simulink model "Quarter_Car"  (R2018b)
settings: Solver=VariableStepAuto  StartTime=0.0  StopTime=60  RelTol=1e-3
values from neighbouring files (symbols this model uses):
  Cs = 100    [Main.m]
  Ct = 0.07    [Main.m]
  Ks = 4000    [Main.m]
  Kt = 7000    [Main.m]
  MR = 0.8    [Main.m]
  Ms = 185    [Main.m]
  Mu = 15    [Main.m]
settings Model: Creator=fcoutu3  LastModifiedBy=katlilee
settings DebuggingCC: LibraryContextMissingDiagnostic=none
settings SFSimCC: SimUseLocalCustomCode=off
settings RTWCC: RTWUseLocalCustomCode=off

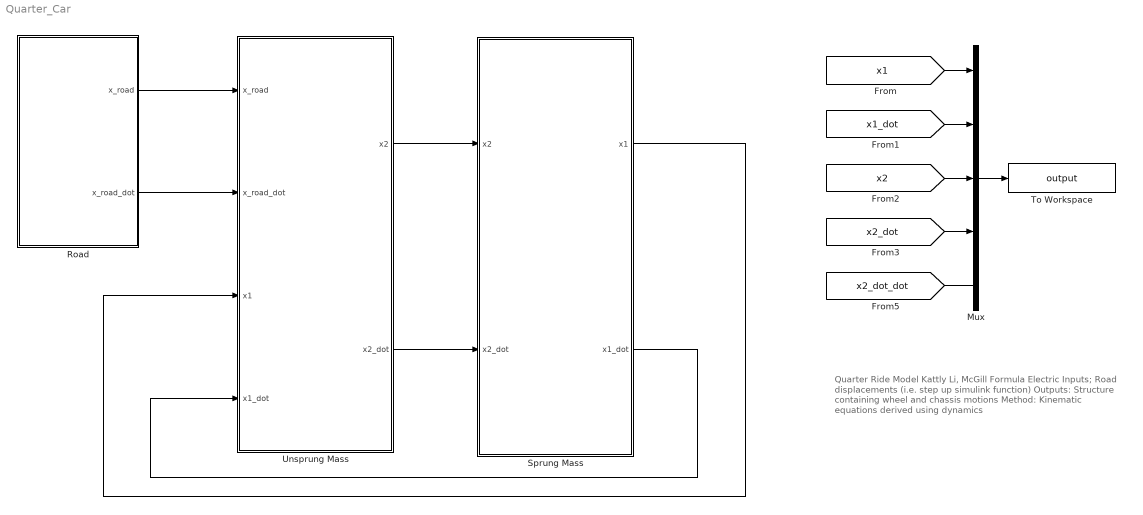
== system Quarter_Car ==
  note: Quarter Ride Model
      | Kattly Li, McGill Formula Electric
      |
      | Inputs;
      | Road displacements
      | (i.e. step up simulink function)
      |
      | Outputs:
      | Structure containing wheel and chassis motions
      |
      | Method:
      | Kinematic equations derived using dynamics
  Mux : Mux  Inputs=5
  Road : Subsystem
  Sprung Mass : Subsystem
  To Workspace : ToWorkspace  VariableName=output  SaveFormat=Structure With Time  SampleTime=-1
  Unsprung Mass : Subsystem
  wires:
  Unsprung Mass/1(x2) -> Sprung Mass/1(x2)
  Sprung Mass/1(x1) -> Unsprung Mass/3(x1)
  Unsprung Mass/2(x2_dot) -> Sprung Mass/2(x2_dot)
  Sprung Mass/2(x1_dot) -> Unsprung Mass/4(x1_dot)
  [x1_dot] -> Mux/2
  [x1] -> Mux/1
  Mux/1 -> To Workspace/1
  [x2] -> Mux/3
  [x2_dot_dot] -> ?
  Road/1(x_road) -> Unsprung Mass/1(x_road)
  Road/2(x_road_dot) -> Unsprung Mass/2(x_road_dot)
  [x2_dot] -> Mux/4

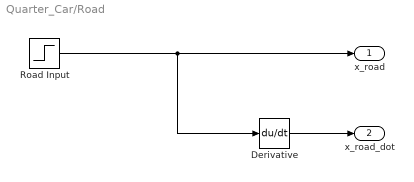
== system Quarter_Car/Road ==
  Derivative : Derivative
  Road Input : Step  After=0.01  SampleTime=0
  x_road : Outport
  x_road_dot : Outport  Port=2
  wires:
  Road Input/1 -> Derivative/1, x_road/1
  Derivative/1 -> x_road_dot/1

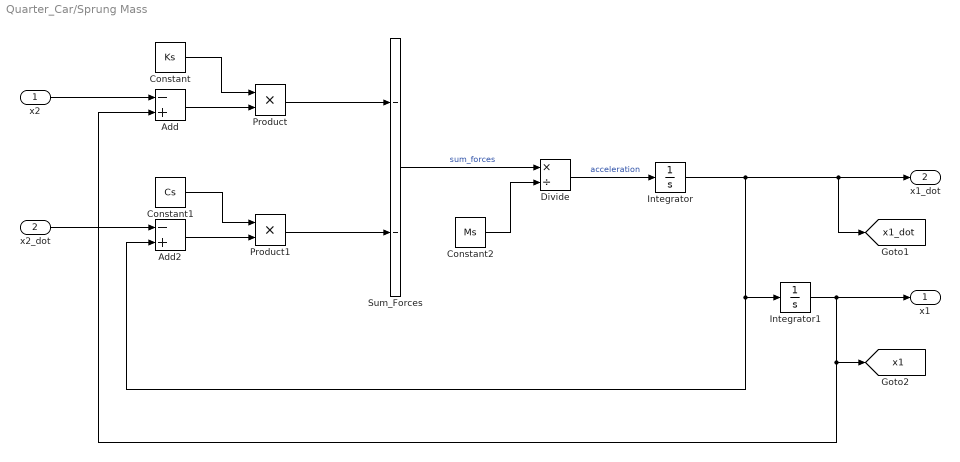
== system Quarter_Car/Sprung Mass ==
  x2 : Inport
  x2_dot : Inport  Port=2
  Add : Sum  Inputs=-+
  Add2 : Sum  Inputs=-+
  Constant : Constant  Value=Ks
  Constant1 : Constant  Value=Cs
  Constant2 : Constant  Value=Ms
  Divide : Product  Inputs=*/
  Integrator : Integrator
  Integrator1 : Integrator
  Product : Product
  Product1 : Product
  Sum_Forces : Sum  Inputs=--
  x1 : Outport
  x1_dot : Outport  Port=2
  tag scope: x1=global, x1_dot=global
  wires:
  Add/1 -> Product/2
  Product/1 -> Sum_Forces/1
  Add2/1 -> Product1/2
  Product1/1 -> Sum_Forces/2
  Constant1/1 -> Product1/1
  Sum_Forces/1 -> Divide/1  "sum_forces"
  Constant2/1 -> Divide/2
  Divide/1 -> Integrator/1  "acceleration"
  Integrator/1 -> x1_dot/1, [x1_dot], Integrator1/1, Add2/2
  Integrator1/1 -> Add/2, [x1], x1/1
  x2/1 -> Add/1
  x2_dot/1 -> Add2/1
  Constant/1 -> Product/1

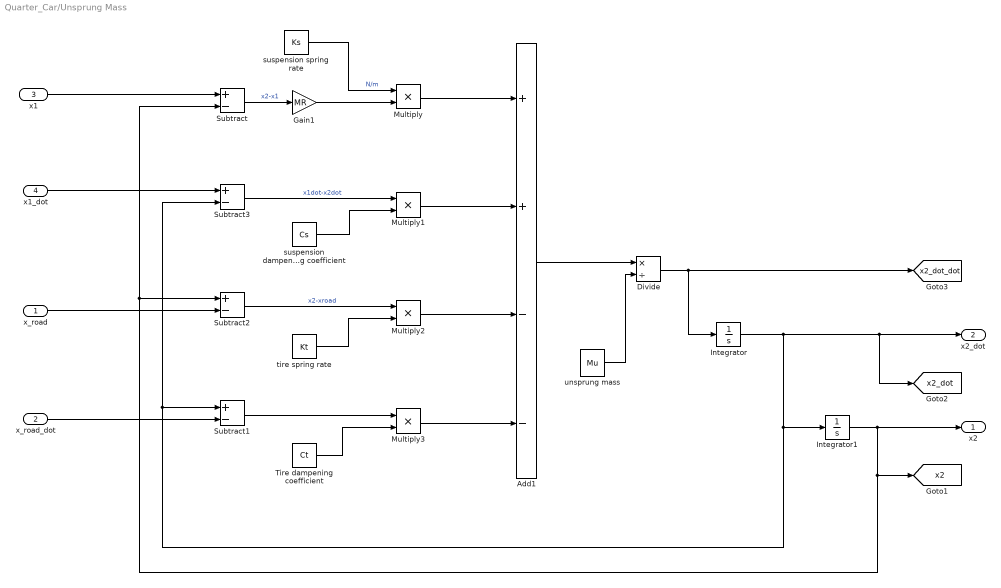
== system Quarter_Car/Unsprung Mass ==
  x_road : Inport
  x_road_dot : Inport  Port=2
  x1 : Inport  Port=3
  x1_dot : Inport  Port=4
  Add1 : Sum  Inputs=++--
  Divide : Product  Inputs=*/
  Gain1 : Gain  Gain=MR
  Integrator : Integrator
  Integrator1 : Integrator
  Multiply{,1..3} (4 alike) : Product
  Subtract{,1..3} (4 alike) : Sum  Inputs=+-
  "Tire dampening coefficient " : Constant  Value=Ct
  "suspension dampening coefficient " : Constant  Value=Cs
  "suspension spring rate " : Constant  Value=Ks
  "tire spring rate " : Constant  Value=Kt
  "unsprung mass " : Constant  Value=Mu
  x2 : Outport
  x2_dot : Outport  Port=2
  tag scope: x2=global, x2_dot=global, x2_dot_dot=global
  wires:
  "suspension spring rate "/1 -> Multiply/1  "N/m"
  Subtract/1 -> Gain1/1  "x2-x1"
  Subtract3/1 -> Multiply1/1  "x1dot-x2dot"
  x1_dot/1 -> Subtract3/1
  Multiply/1 -> Add1/1
  Multiply1/1 -> Add1/2
  "suspension dampening coefficient "/1 -> Multiply1/2
  x1/1 -> Subtract/1
  x_road/1 -> Subtract2/2
  x_road_dot/1 -> Subtract1/2
  Subtract2/1 -> Multiply2/1  "x2-xroad"
  "Tire dampening coefficient "/1 -> Multiply3/2
  Subtract1/1 -> Multiply3/1
  Multiply2/1 -> Add1/3
  Multiply3/1 -> Add1/4
  "unsprung mass "/1 -> Divide/2
  Add1/1 -> Divide/1
  Divide/1 -> [x2_dot_dot], Integrator/1
  Integrator/1 -> Subtract3/2, Subtract1/1, Integrator1/1, [x2_dot], x2_dot/1
  Integrator1/1 -> x2/1, Subtract/2, Subtract2/1, [x2]
  Gain1/1 -> Multiply/2
  "tire spring rate "/1 -> Multiply2/2
